simulink library "TrgtPosSelcLib"  (R2018b)
settings: Solver=VariableStepAuto  StartTime=0.0  StopTime=10.0  RelTol=1e-3
settings Model: Creator=sn2xws  LastModifiedBy=sn2xws

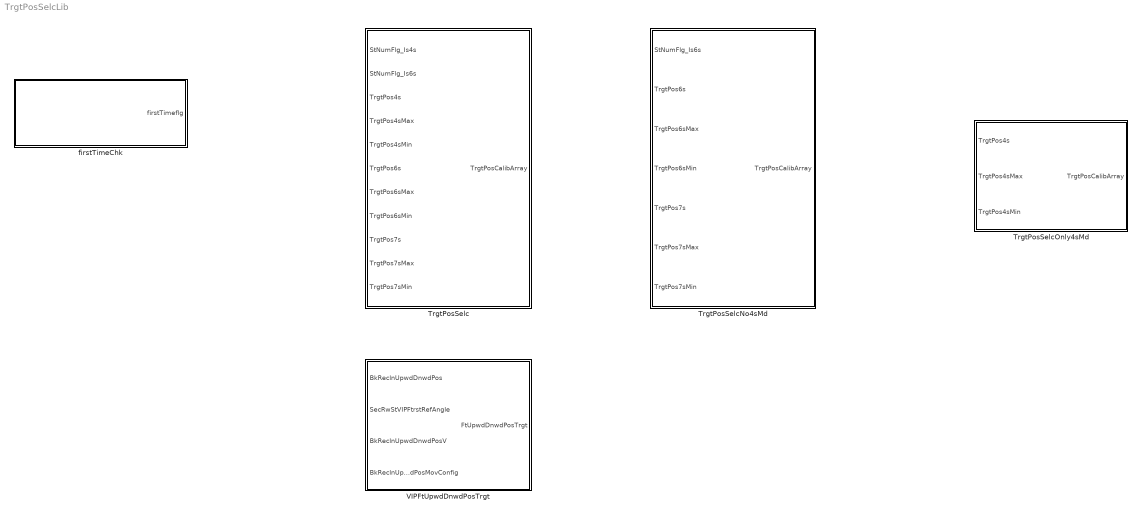
== system TrgtPosSelcLib ==
  TrgtPosSelc : Subsystem
  TrgtPosSelcNo4sMd : Subsystem
  TrgtPosSelcOnly4sMd : Subsystem
  VIPFtUpwdDnwdPosTrgt : Subsystem
  firstTimeChk : Stateflow chart  TreatAsAtomicUnit=on

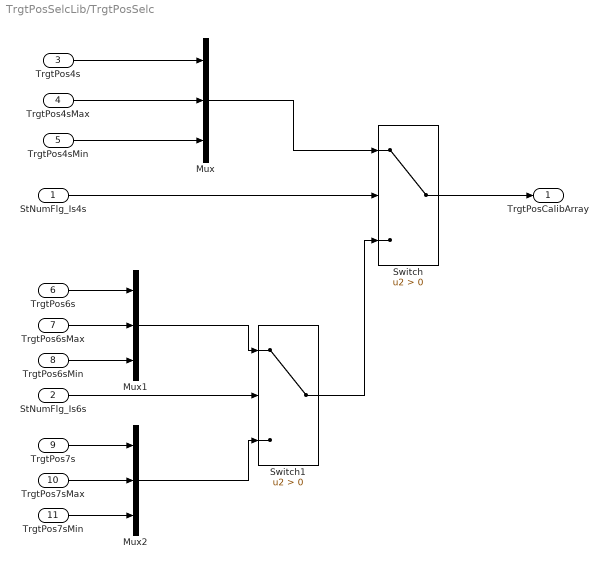
== system TrgtPosSelcLib/TrgtPosSelc ==
  StNumFlg_Is4s : Inport
  StNumFlg_Is6s : Inport  Port=2
  TrgtPos4s : Inport  Port=3
  TrgtPos4sMax : Inport  Port=4
  TrgtPos4sMin : Inport  Port=5
  TrgtPos6s : Inport  Port=6
  TrgtPos6sMax : Inport  Port=7
  TrgtPos6sMin : Inport  Port=8
  TrgtPos7s : Inport  Port=9
  TrgtPos7sMax : Inport  Port=10
  TrgtPos7sMin : Inport  Port=11
  Mux : Mux  Inputs=3
  Mux1 : Mux  Inputs=3
  Mux2 : Mux  Inputs=3
  Switch : Switch  Criteria=u2 > Threshold
  Switch1 : Switch  Criteria=u2 > Threshold
  TrgtPosCalibArray : Outport
      settings: EnsureOutportIsVirtual=on
  wires:
  TrgtPos4sMax/1 -> Mux/2
  TrgtPos4sMin/1 -> Mux/3
  TrgtPos6sMin/1 -> Mux1/3
  StNumFlg_Is4s/1 -> Switch/2
  TrgtPos7sMin/1 -> Mux2/3
  Mux1/1 -> Switch1/1
  Mux/1 -> Switch/1
  TrgtPos4s/1 -> Mux/1
  TrgtPos6sMax/1 -> Mux1/2
  TrgtPos7s/1 -> Mux2/1
  Switch1/1 -> Switch/3
  Mux2/1 -> Switch1/3
  TrgtPos6s/1 -> Mux1/1
  TrgtPos7sMax/1 -> Mux2/2
  StNumFlg_Is6s/1 -> Switch1/2
  Switch/1 -> TrgtPosCalibArray/1

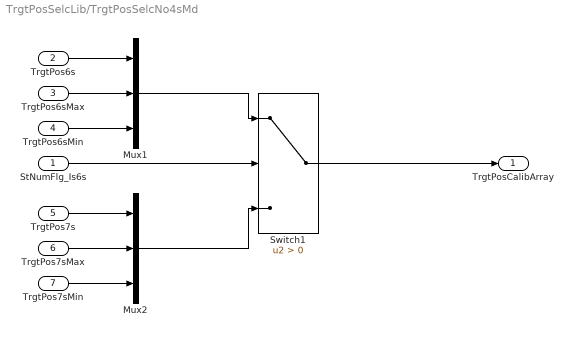
== system TrgtPosSelcLib/TrgtPosSelcNo4sMd ==
  StNumFlg_Is6s : Inport
  TrgtPos6s : Inport  Port=2
  TrgtPos6sMax : Inport  Port=3
  TrgtPos6sMin : Inport  Port=4
  TrgtPos7s : Inport  Port=5
  TrgtPos7sMax : Inport  Port=6
  TrgtPos7sMin : Inport  Port=7
  Mux1 : Mux  Inputs=3
  Mux2 : Mux  Inputs=3
  Switch1 : Switch  Criteria=u2 > Threshold
  TrgtPosCalibArray : Outport
      settings: EnsureOutportIsVirtual=on
  wires:
  TrgtPos6sMin/1 -> Mux1/3
  TrgtPos7sMin/1 -> Mux2/3
  Mux1/1 -> Switch1/1
  TrgtPos6sMax/1 -> Mux1/2
  TrgtPos7s/1 -> Mux2/1
  Mux2/1 -> Switch1/3
  TrgtPos6s/1 -> Mux1/1
  TrgtPos7sMax/1 -> Mux2/2
  StNumFlg_Is6s/1 -> Switch1/2
  Switch1/1 -> TrgtPosCalibArray/1

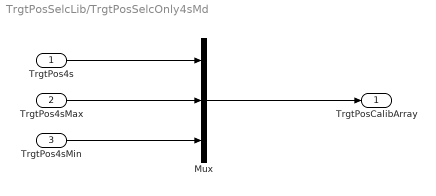
== system TrgtPosSelcLib/TrgtPosSelcOnly4sMd ==
  TrgtPos4s : Inport
  TrgtPos4sMax : Inport  Port=2
  TrgtPos4sMin : Inport  Port=3
  Mux : Mux  Inputs=3
  TrgtPosCalibArray : Outport
      settings: EnsureOutportIsVirtual=on
  wires:
  TrgtPos4s/1 -> Mux/1
  TrgtPos4sMax/1 -> Mux/2
  TrgtPos4sMin/1 -> Mux/3
  Mux/1 -> TrgtPosCalibArray/1

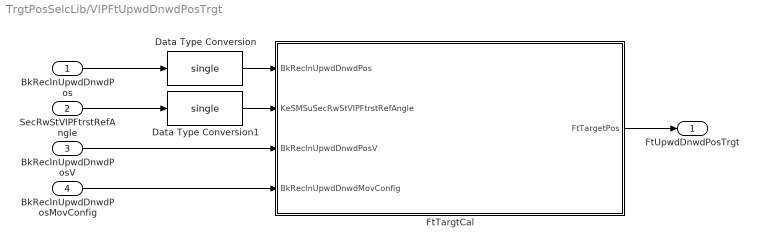
== system TrgtPosSelcLib/VIPFtUpwdDnwdPosTrgt ==
  BkReclnUpwdDnwdPos : Inport
  SecRwStVIPFtrstRefAngle : Inport  Port=2
  BkReclnUpwdDnwdPosV : Inport  Port=3
  BkReclnUpwdDnwdPosMovConfig : Inport  Port=4
  Data Type Conversion : DataTypeConversion  OutDataTypeStr=single
  Data Type Conversion1 : DataTypeConversion  OutDataTypeStr=single
  FtTargtCal : Stateflow chart  TreatAsAtomicUnit=on
  FtUpwdDnwdPosTrgt : Outport
  wires:
  SecRwStVIPFtrstRefAngle/1 -> Data Type Conversion1/1
  Data Type Conversion/1 -> FtTargtCal/1(BkReclnUpwdDnwdPos)
  Data Type Conversion1/1 -> FtTargtCal/2(KeSMSuSecRwStVIPFtrstRefAngle)
  FtTargtCal/1(FtTargetPos) -> FtUpwdDnwdPosTrgt/1
  BkReclnUpwdDnwdPos/1 -> Data Type Conversion/1
  BkReclnUpwdDnwdPosV/1 -> FtTargtCal/3(BkReclnUpwdDnwdPosV)
  BkReclnUpwdDnwdPosMovConfig/1 -> FtTargtCal/4(BkReclnUpwdDnwdMovConfig)

== stateflow chart TrgtPosSelcLib/firstTimeChk ==
  (default) -> (junction 1)
  (junction 1) -> (junction 5) [order 1] : [chkflg ==0]
  (junction 1) -> (junction 3) [order 2] : {firstTimeflg = 0;}
  (junction 5) -> (junction 7) : {firstTimeflg = 1;
      | chkflg=1;}
  (junction 7) -> (junction 3)
  (junction 3) -> (junction 10)
  data: chkflg local boolean size=1; firstTimeflg output boolean size=1

== stateflow chart TrgtPosSelcLib/VIPFtUpwdDnwdPosTrgt/FtTargtCal ==
  (default) -> (junction 36)
  (junction 36) -> (junction 38) [order 1] : [BkReclnUpwdDnwdPosV ||!BkReclnUpwdDnwdMovConfig]
  (junction 38) -> (junction 40) : {BkReclnUpwdDnwdPostmp=0;}
  (junction 36) -> (junction 4) [order 2] : {BkReclnUpwdDnwdPostmp = BkReclnUpwdDnwdPos;}
  (junction 40) -> (junction 4)
  (junction 4) -> (junction 6) : {
      | FtTargetAngle = KeSMSuSecRwStVIPFtrstRefAngle-BkReclnUpwdDnwdPostmp/4000*78;
      | }
  (junction 6) -> (junction 9) [order 1] : [FtTargetAngle<0]
  (junction 6) -> (junction 13) [order 2]
  (junction 9) -> (junction 11) : {
      | FtTargetAngle=0;
      | }
  (junction 11) -> (junction 13)
  (junction 13) -> (junction 16)
  (junction 16) -> (junction 18) [order 1] : [FtTargetAngle>=108.2216]
  (junction 16) -> (junction 25) [order 2] : {
      | n=(sqrt(26933.84-(cos(FtTargetAngle*3.14159/180+0.43)*8110))-139.91)/0.12;
      | }
  (junction 18) -> (junction 20) : {
      | FtTargetPos=4000;
      | }
  (junction 25) -> (junction 28) : {
      | tmpTargetPos = n*4000;
      | tmpTargetPos = tmpTargetPos/335.245;
      | FtTargetPos = tmpTargetPos;
      | }
  (junction 20) -> (junction 28)
  (junction 28) -> (junction 32)
  data: BkReclnUpwdDnwdPos input single; KeSMSuSecRwStVIPFtrstRefAngle input single; FtTargetPos output uint16; FtTargetAngle local single; n local single; tmpTargetPos local single; BkReclnUpwdDnwdPosV input boolean; BkReclnUpwdDnwdMovConfig input boolean; BkReclnUpwdDnwdPostmp local single
